simulink model "model_sim"  (R2016a)
settings: Solver=ode4  StartTime=0.0  StopTime=40  FixedStep=0.01  RelTol=1e-3
values from neighbouring files (symbols this model uses):
  K = X0(1)    [cel.m]    (also in cel_t.m; lsm.m = par(1); lsm_tarcie.m = par(1))
  T = X0(2)    [cel.m]    (also in cel_t.m; lsm.m = par(2); lsm_tarcie.m = par(2))
  tau = X0(3)    [cel.m]    (also in cel_t.m; lsm.m = par(3); lsm_tarcie.m = par(3))
settings Model: Creator=Maciek  LastModifiedBy=Maciek

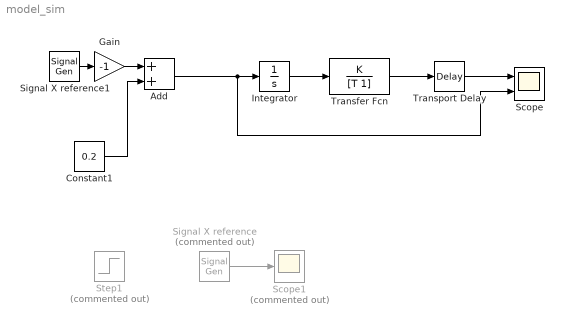
== system model_sim ==
  Add : Sum
  Constant1 : Constant  Value=0.2
  Gain : Gain  Gain=-1
  Integrator : Integrator
  Scope : Scope  NumInputPorts=2
  Scope1 : Scope  Commented=on
  Signal X reference : SignalGenerator  Commented=on  WaveForm=sawtooth  Amplitude=0.02  Frequency=0.06
  Signal X reference1 : SignalGenerator  WaveForm=sawtooth  Amplitude=0.2  Frequency=0.02
  Step1 : Step  Commented=on  Time=20  After=-1  SampleTime=0
  Transfer Fcn : TransferFcn  Numerator=K  Denominator=[T 1]
  Transport Delay : TransportDelay  DelayTime=tau
  wires:
  Integrator/1 -> Transfer Fcn/1
  Constant1/1 -> Add/2
  Signal X reference/1 -> Scope1/1
  Transfer Fcn/1 -> Transport Delay/1
  Add/1 -> Scope/2, Integrator/1
  Signal X reference1/1 -> Gain/1
  Gain/1 -> Add/1
  Transport Delay/1 -> Scope/1
